simulink model "translatorische_Windscherung"  (R2020b)
settings: Solver=VariableStepAuto  StartTime=0.0  StopTime=10.0  RelTol=1e-3
settings Model: Creator=Dogukan  LastModifiedBy=Dogukan

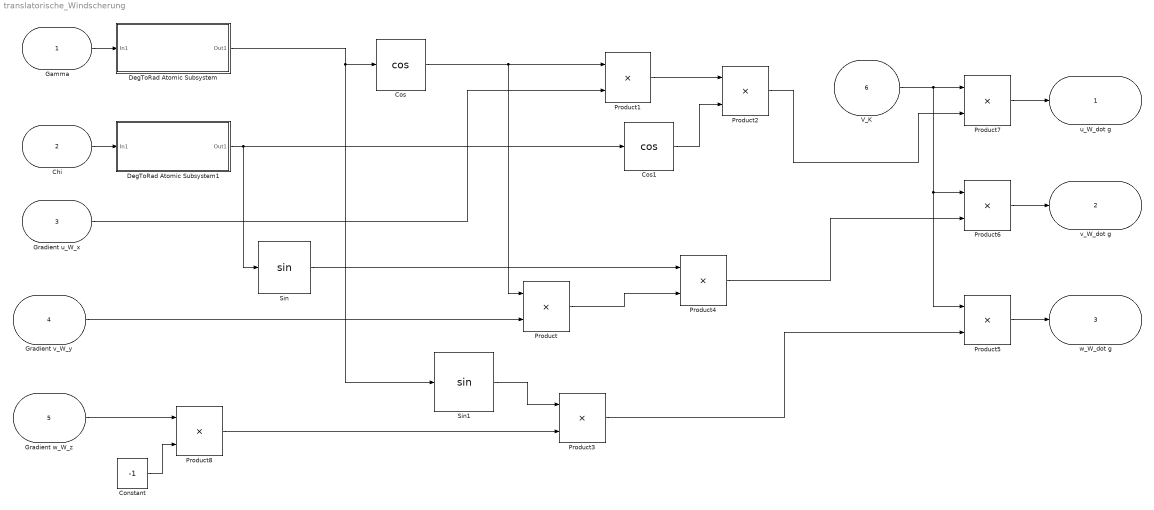
== system translatorische_Windscherung ==
  Gamma : Inport
  Chi : Inport  Port=2
  Gradient u_W_x : Inport  Port=3
  Gradient v_W_y : Inport  Port=4
  Gradient w_W_z : Inport  Port=5
  V_K : Inport  Port=6
  Constant : Constant  Value=-1
  Cos : Trigonometry  Operator=cos
  Cos1 : Trigonometry  Operator=cos
  DegToRad Atomic Subsystem : Subsystem  TreatAsAtomicUnit=on
  DegToRad Atomic Subsystem1 : Subsystem  TreatAsAtomicUnit=on
  Product{,1..8} (9 alike) : Product
  Sin : Trigonometry
  Sin1 : Trigonometry
  u_W_dot g : Outport
  v_W_dot g : Outport  Port=2
  w_W_dot g : Outport  Port=3
  wires:
  Gamma/1 -> DegToRad Atomic Subsystem/1(In1)
  DegToRad Atomic Subsystem/1(Out1) -> Cos/1, Sin1/1
  V_K/1 -> Product5/1, Product6/1, Product7/1
  Product5/1 -> w_W_dot g/1
  Product6/1 -> v_W_dot g/1
  Product7/1 -> u_W_dot g/1
  Gradient w_W_z/1 -> Product8/1
  Constant/1 -> Product8/2
  Product8/1 -> Product3/2
  Sin1/1 -> Product3/1
  Chi/1 -> DegToRad Atomic Subsystem1/1(In1)
  Gradient u_W_x/1 -> Product1/2
  Cos/1 -> Product1/1, Product/1
  DegToRad Atomic Subsystem1/1(Out1) -> Cos1/1, Sin/1
  Cos1/1 -> Product2/2
  Product1/1 -> Product2/1
  Product2/1 -> Product7/2
  Gradient v_W_y/1 -> Product/2
  Product/1 -> Product4/2
  Sin/1 -> Product4/1
  Product4/1 -> Product6/2
  Product3/1 -> Product5/2

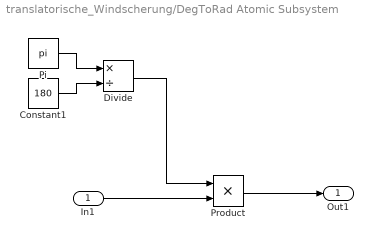
== system translatorische_Windscherung/DegToRad Atomic Subsystem ==
  In1 : Inport
  Constant1 : Constant  Value=180
  Divide : Product  Inputs=*/
  Pi : Constant  Value=pi  OutDataTypeStr=Inherit: Inherit via back propagation
  Product : Product
  Out1 : Outport
  wires:
  Pi/1 -> Divide/1
  Constant1/1 -> Divide/2
  Divide/1 -> Product/1
  In1/1 -> Product/2
  Product/1 -> Out1/1

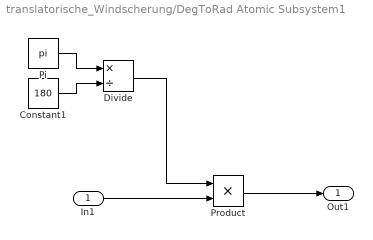
== system translatorische_Windscherung/DegToRad Atomic Subsystem1 ==
  In1 : Inport
  Constant1 : Constant  Value=180
  Divide : Product  Inputs=*/
  Pi : Constant  Value=pi  OutDataTypeStr=Inherit: Inherit via back propagation
  Product : Product
  Out1 : Outport
  wires:
  Pi/1 -> Divide/1
  Constant1/1 -> Divide/2
  Divide/1 -> Product/1
  In1/1 -> Product/2
  Product/1 -> Out1/1
